simulink model "ES100A_SysStMod"  (R2013b)
settings: Solver=ode45  StartTime=0.0  StopTime=10  FixedStep=0.002  RelTol=1e-3
undefined symbols (not defined in the file): ELECGLBPRM_STRTUPSTTMPLMONININTESTCMPL_CNT_U08, sigbuilder_block, SysSt1, SYSSTMODPRSNTSTDI_CNT_U16, SYSSTMODPRSNTSTENA_CNT_U16, SYSSTMODPRSNTSTOFF_CNT_U16, SYSSTMODPRSNTSTWRMININ_CNT_U16
libraries: simulink x2
settings Model: Creator=pz79n7  LastModifiedBy=nzg49t
settings Model: ModifiedHistory=|
  | 05JN13: ES-10B Revision 011.  Added PStep/NStep counter (shown in red)
  | and calibrations to support.  This is in the block entitled "Safety Check" and
  | impacts NTC 0CB.  This change is in support of anomaly #5108.
  | 
  | 01JL13: ES-10B Revision 012.  Added note inside block "Determine Next State"
  | to clearly indicate that the state of the TOD signal is to be logic LOW when
  | switching is stopped.
  | 
  | 25JA15: ES-10B Revision 014 - Added links from Model to the FR document
  | 
  | 25JA15: ES-10B Revision 015 - Removed redundant check logic as it is no longer
  | needed based on new shutdown design placed into ES-34B.  Removed output
  | SysCSystemState and NTC 0CB.
settings DataIOCC: SignalLoggingSaveFormat=ModelDataLogs
settings OptimizationCC: ExpressionDepthLimit=2147483647
settings DebuggingCC: FcnCallInpInsideContextMsg=UseLocalSettings  StateNameClashWarn=warning
settings GRTTargetCC: CombineOutputUpdateFcns=off  GRTInterface=on

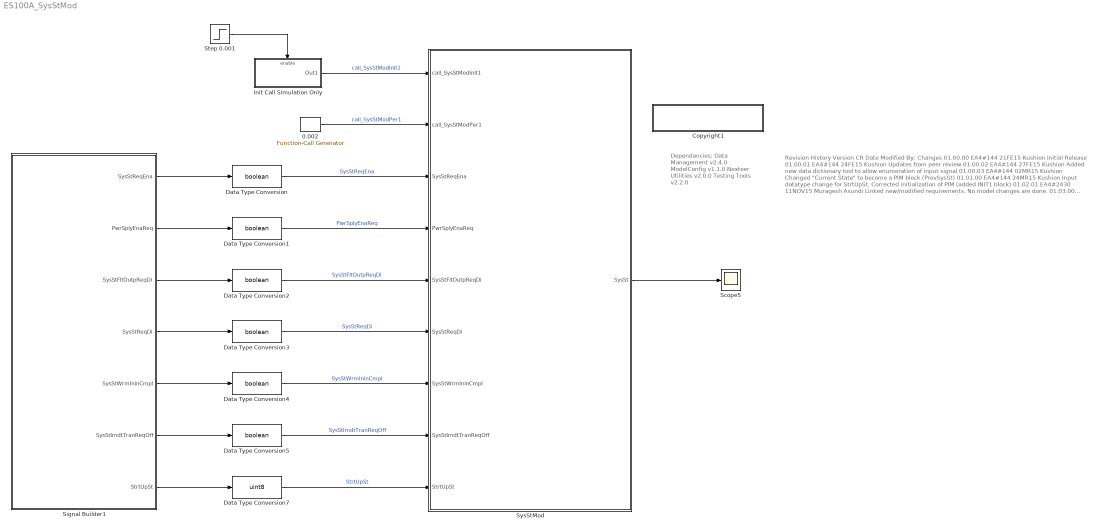
== system ES100A_SysStMod ==
  note: Revision History
      |
      | Version		CR			Date 		Modified By: 		Changes
      | 01.00.00 	EA4#144	21FE15		Kushion			Initial Release
      | 01.00.01		EA4#144       24FE15		Kushion			Updates from peer review
      | 01.00.02        EA4#144	27FE15		Kushion			Added new data dictionary tool to allow enumeration of input signal
      | 01.00.03		EA4#144	02MR15		Kushion			Changed "Current State" to become a PIM block (PrevSysSt)
      | 01.01.00	       EA4#144       24MR15        Kushion                 Input datatype change for StrtUpSt.  Corrected initialization of PIM (added INIT1 block)
      | 01.02.01        EA4#2430     11NOV15     Muragesh Asundi   Linked new/modified requirements. No model changes are done.
      | 01.03.00		EA4#4826	31MAR16	Kumaraswamy	Updated SysStReqEn => SysStReqEna, PwrSplyEnReq=> PwrSplyEnaReq to comply with
      | 													AUTOSAR Naming convention
  note: Dependancies:
      |    Data Management v2.4.0
      |    ModelConfig v1.1.0
      |    Nexteer Utilities v2.0.0
      |    Testing Tools v2.2.0
  0.002 : simulink/Ports & Subsystems/Function-Call Generator  sample_time=0.002  numberOfIterations=1
  Copyright1 : Subsystem  Description=|  mask(Copyright Information){none=on}
      | Copyright info block.                                               
      |                                                                     
      | Place copyright information at the top of every subsystem in design.
      mask prompts: none "No parameters"
      mask help: Place copyright information at the top of every subsystem in design.
      mask Display:
      | NxtrConf = 'Nexteer Confidential';
      | 
      | sys = bdroot; %handle for the current model ("system")
      | first = get_param(sys,'Created');
      | if(isempty(first))
      |     first = datestr(now,'yyyy');
      | else
      |     first = first(end-3:end);  %year is last four digits
      | end
      | 
      | last = get_param(sys,'LastModifiedDate');
      | if isempty(last)
      |     last = datestr(now,'yyyy');
      | else
      |     last = last(end-3:end);
      | end
      | 
      | if strcmp(first,last)
      |     fprintf('%s\nCopyright  %s Nexteer',NxtrConf,first);
      | else
      |     fprintf('%s\n%s%s-%s Nexteer',NxtrConf,char(169),first,last);
      | end
  Data Type Conversion : DataTypeConversion  Priority=1  OutDataTypeStr=boolean
  Data Type Conversion1 : DataTypeConversion  Priority=2  OutDataTypeStr=boolean
  Data Type Conversion2 : DataTypeConversion  Priority=3  OutDataTypeStr=boolean
  Data Type Conversion3 : DataTypeConversion  Priority=4  OutDataTypeStr=boolean
  Data Type Conversion4 : DataTypeConversion  Priority=5  OutDataTypeStr=boolean
  Data Type Conversion5 : DataTypeConversion  OutDataTypeStr=boolean
  Data Type Conversion7 : DataTypeConversion  OutDataTypeStr=uint8
  Init Call Simulation Only : Subsystem  TreatAsAtomicUnit=on
  Scope5 : Scope
      settings: TimeRange=10  YMin=-1  SaveName=ScopeData5  MaxDataPoints=10000
  Signal Builder1 : Subsystem  Tag=STV Subsys  LoadFcn=sigbuilder_block('load');  StartFcn=sigbuilder_block('start');  StopFcn=sigbuilder_block('stop');  ClipboardFcn=sigbuilder_block('clipboard');  mask(Sigbuilder block){}
      mask help: Create and generate interchangeable groups of signals whose waveforms are piecewise linear.
      mask init:
      | if ~strcmp(get_param(bdroot(gcbh),'SimulationStatus'),'stopped') tuvar = sigbuilder_block('maskInit'); end
      settings: CopyFcn=sigbuilder_block('copy');  DeleteFcn=sigbuilder_block('delete');  ModelCloseFcn=sigbuilder_block('modelClose');  PreSaveFcn=sigbuilder_block('preSave');  PauseFcn=sigbuilder_block('pause')  ContinueFcn=sigbuilder_block('continue')  NameChangeFcn=sigbuilder_block('namechange');  OpenFcn=sigbuilder_block('open',[1464 -138.75 381 502.5 ]);  CloseFcn=sigbuilder_block('close');
      mask Display: plot(0,0,100,100,[10,10,40,40,10],[80,20,20,80,80],[40,10],[50,50], [40,27,10],[65,72,56],[40,25,25,10],[28,28,43,43]);
  Step 0.001 : Step  Time=0.001  Before=1  After=0  SampleTime=0
  SysStMod : Subsystem  RequirementInfo={'linktype_rmi_doors' '0000cf67 (/E-STEER Core/SubSystem Specifications/Electrical Actuator/Control Module/FDD Module Requirements/EA4/ES100A_SysStMod_1)' '#ES100A_72' 'true' 'REQ: ES100A_72' '' ; 'linktype_rmi_doors' '0000cf67 (/E-STEER Core/SubSystem Specifications/Electrical Actuator/Control Module/FDD Module Requirements/EA4/ES100A_SysStMod_1)' '#ES100A_80' 'true' 'REQ: ES100A_80' '' } %GIDa_7525e75c_09f9_4f81_91ae_9ba7a4b2fbd2
  wires:
  SysStMod/1(SysSt) -> Scope5/1
  Signal Builder1/1(SysStReqEna) -> Data Type Conversion/1
  Signal Builder1/2(PwrSplyEnaReq) -> Data Type Conversion1/1
  Signal Builder1/3(SysStFltOutpReqDi) -> Data Type Conversion2/1
  Signal Builder1/4(SysStReqDi) -> Data Type Conversion3/1
  Signal Builder1/5(SysStWrmIninCmpl) -> Data Type Conversion4/1
  Signal Builder1/6(SysStImdtTranReqOff) -> Data Type Conversion5/1
  Data Type Conversion/1 -> SysStMod/3(SysStReqEna)  "SysStReqEna"
  Data Type Conversion1/1 -> SysStMod/4(PwrSplyEnaReq)  "PwrSplyEnaReq"
  Data Type Conversion2/1 -> SysStMod/5(SysStFltOutpReqDi)  "SysStFltOutpReqDi"
  Data Type Conversion3/1 -> SysStMod/6(SysStReqDi)  "SysStReqDi"
  Data Type Conversion4/1 -> SysStMod/7(SysStWrmIninCmpl)  "SysStWrmIninCmpl"
  Data Type Conversion5/1 -> SysStMod/8(SysStImdtTranReqOff)  "SysStImdtTranReqOff"
  Signal Builder1/7(StrtUpSt) -> Data Type Conversion7/1
  0.002/1 -> SysStMod/2(call_SysStModPer1)  "call_SysStModPer1"
  Data Type Conversion7/1 -> SysStMod/9(StrtUpSt)  "StrtUpSt"
  Init Call Simulation Only/1(Out1) -> SysStMod/1(call_SysStModInit1)  "call_SysStModInit1"
  Step 0.001/1 -> Init Call Simulation Only/Enable

== system ES100A_SysStMod/Copyright1 ==

== system ES100A_SysStMod/Init Call Simulation Only ==
  Enable : EnablePort
  0.001 : simulink/Ports & Subsystems/Function-Call Generator  sample_time=0.001  numberOfIterations=1
  Out1 : Outport
  wires:
  0.001/1 -> Out1/1

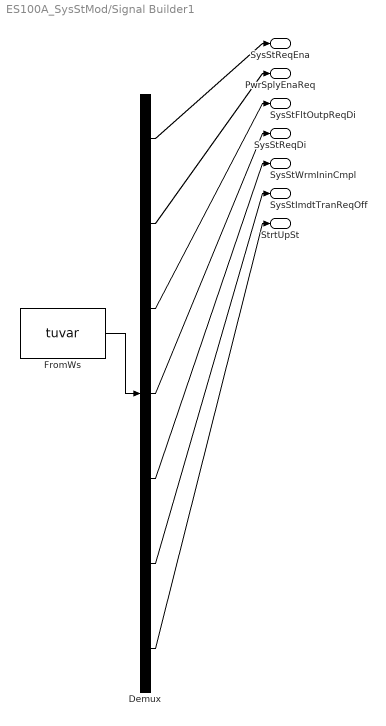
== system ES100A_SysStMod/Signal Builder1 ==
  Demux : Demux  Tag=STV Demux  Outputs=7
  FromWs : FromWorkspace  Tag=STV FromWs  VariableName=tuvar  SampleTime=0.002
      SigBuilderData=|
      | common.afterFinalStr = 'Extrapolate'
      | common.sampleTime = '0.002'
      | dataSet(1).timeRange = [0 10]
      | dataSet(1).name = 'Normal Start up to Enable'
      | dataSet(2).timeRange = [0 10]
      | dataSet(2).name = 'Confirm no ENABLE until WI is complete'
      | dataSet(3).timeRange = [0 10]
      | dataSet(3).name = 'Normal cycle - WI, Operate, Disable, OFF'
      | dataSet(4).timeRange = [0 10]
      | dataSet(4).name = 'While in WI, Change ReqDI, no changem Cgange Fault, DIS'
      | dataSet(5).timeRange = [0 10]
      | dataSet(5).name = 'Rapid shutdown while in operate state'
      | dataSet(6).timeRange = [0 10]
      | dataSet(6).name = 'Quick Ignition (assumed prior to TOD off)'
      | dataSet(7).timeRange = [0 10]
      | dataSet(7).name = 'Failure in warm init prior to temporal monitor completing'
      | dataSet(8).timeRange = [0 10]
      | dataSet(8).name = 'Immediate request from Reset or FBL'
      | sbobj.Groups(1).Name = 'Normal Start up to Enable'
      | sbobj.Groups(1).Signals(1).Name = 'SysStReqEna'
      | sbobj.Groups(1).Signals(1).XData = [0 2 2 6 6 10]
      | sbobj.Groups(1).Signals(1).YData = [0 0 1 1 0 0]
      | sbobj.Groups(1).Signals(2).Name = 'PwrSplyEnaReq'
      | sbobj.Groups(1).Signals(2).XData = [0 6 6 10]
      | sbobj.Groups(1).Signals(2).YData = [1 1 0 0]
      | sbobj.Groups(1).Signals(3).Name = 'SysStFltOutpReqDi'
      | sbobj.Groups(1).Signals(3).XData = [0 4 6 10]
      | sbobj.Groups(1).Signals(3).YData = [0 0 0 0]
      | sbobj.Groups(1).Signals(4).Name = 'SysStReqDi'
      | sbobj.Groups(1).Signals(4).XData = [0 4 6 10]
      | sbobj.Groups(1).Signals(4).YData = [0 0 0 0]
      | sbobj.Groups(1).Signals(5).Name = 'SysStWrmIninCmpl'
      | sbobj.Groups(1).Signals(5).XData = [0 1 1 6 6 10]
      | sbobj.Groups(1).Signals(5).YData = [0 0 1 1 0 0]
      | sbobj.Groups(1).Signals(6).Name = 'SysStImdtTranReqOff'
      | sbobj.Groups(1).Signals(6).XData = [0 4 6 10]
      | sbobj.Groups(1).Signals(6).YData = [0 0 0 0]
      | sbobj.Groups(1).Signals(7).Name = 'StrtUpSt'
      | sbobj.Groups(1).Signals(7).XData = [0 0.5 0.5 6 6 10]
      | sbobj.Groups(1).Signals(7).YData = [1 1 3 3 1 1]
      | sbobj.Groups(2).Name = 'Confirm no ENABLE until WI is complete'
      | sbobj.Groups(2).Signals(1).Name = 'SysStReqEna'
      | sbobj.Groups(2).Signals(1).XData = [0 0.5 0.5 6 6 10]
      | sbobj.Groups(2).Signals(1).YData = [0 0 1 1 0 0]
      | sbobj.Groups(2).Signals(2).Name = 'PwrSplyEnaReq'
      | sbobj.Groups(2).Signals(2).XData = [0 6 6 10]
      | sbobj.Groups(2).Signals(2).YData = [1 1 0 0]
      | sbobj.Groups(2).Signals(3).Name = 'SysStFltOutpReqDi'
      | sbobj.Groups(2).Signals(3).XData = [0 4 6 10]
      | sbobj.Groups(2).Signals(3).YData = [0 0 0 0]
      | sbobj.Groups(2).Signals(4).Name = 'SysStReqDi'
      | sbobj.Groups(2).Signals(4).XData = [0 8 8 10]
      | sbobj.Groups(2).Signals(4).YData = [0 0 1 1]
      | sbobj.Groups(2).Signals(5).Name = 'SysStWrmIninCmpl'
      | sbobj.Groups(2).Signals(5).XData = [0 1 1 6 6 10]
      | sbobj.Groups(2).Signals(5).YData = [0 0 1 1 0 0]
      | sbobj.Groups(2).Signals(6).Name = 'SysStImdtTranReqOff'
      | sbobj.Groups(2).Signals(6).XData = [0 4 6 10]
      | sbobj.Groups(2).Signals(6).YData = [0 0 0 0]
      | sbobj.Groups(2).Signals(7).Name = 'StrtUpSt'
      | sbobj.Groups(2).Signals(7).XData = [0 0.5 0.5 6 6 10]
      | sbobj.Groups(2).Signals(7).YData = [1 1 3 3 1 1]
      | sbobj.Groups(3).Name = 'Normal cycle - WI, Operate, Disable, OFF'
      | sbobj.Groups(3).Signals(1).Name = 'SysStReqEna'
      | sbobj.Groups(3).Signals(1).XData = [0 2 2 6 6 10]
      | sbobj.Groups(3).Signals(1).YData = [0 0 1 1 0 0]
      | sbobj.Groups(3).Signals(2).Name = 'PwrSplyEnaReq'
      | sbobj.Groups(3).Signals(2).XData = [0 9 9 10]
      | sbobj.Groups(3).Signals(2).YData = [1 1 0 0]
      | sbobj.Groups(3).Signals(3).Name = 'SysStFltOutpReqDi'
      | sbobj.Groups(3).Signals(3).XData = [0 7.5 10]
      | sbobj.Groups(3).Signals(3).YData = [0 0 0]
      | sbobj.Groups(3).Signals(4).Name = 'SysStReqDi'
      | sbobj.Groups(3).Signals(4).XData = [0 7.5 7.5 10]
      | sbobj.Groups(3).Signals(4).YData = [0 0 1 1]
      | sbobj.Groups(3).Signals(5).Name = 'SysStWrmIninCmpl'
      | sbobj.Groups(3).Signals(5).XData = [0 1 1 10]
      | sbobj.Groups(3).Signals(5).YData = [0 0 1 1]
      | sbobj.Groups(3).Signals(6).Name = 'SysStImdtTranReqOff'
      | sbobj.Groups(3).Signals(6).XData = [0 4 6 10]
      | sbobj.Groups(3).Signals(6).YData = [0 0 0 0]
      | sbobj.Groups(3).Signals(7).Name = 'StrtUpSt'
      | sbobj.Groups(3).Signals(7).XData = [0 0.5 0.5 10]
      | sbobj.Groups(3).Signals(7).YData = [1 1 3 3]
      | sbobj.Groups(4).Name = 'While in WI, Change ReqDI, no changem Cgange Fault, DIS'
      | sbobj.Groups(4).Signals(1).Name = 'SysStReqEna'
      | sbobj.Groups(4).Signals(1).XData = [0 3 10]
      | sbobj.Groups(4).Signals(1).YData = [0 0 0]
      | sbobj.Groups(4).Signals(2).Name = 'PwrSplyEnaReq'
      | sbobj.Groups(4).Signals(2).XData = [0 9 9 10]
      | sbobj.Groups(4).Signals(2).YData = [1 1 0 0]
      | sbobj.Groups(4).Signals(3).Name = 'SysStFltOutpReqDi'
      | sbobj.Groups(4).Signals(3).XData = [0 5 5 10]
      | sbobj.Groups(4).Signals(3).YData = [0 0 1 1]
      | sbobj.Groups(4).Signals(4).Name = 'SysStReqDi'
      | sbobj.Groups(4).Signals(4).XData = [0 3 3 10]
      | sbobj.Groups(4).Signals(4).YData = [0 0 1 1]
      | sbobj.Groups(4).Signals(5).Name = 'SysStWrmIninCmpl'
      | sbobj.Groups(4).Signals(5).XData = [0 1 1 10]
      | sbobj.Groups(4).Signals(5).YData = [0 0 1 1]
      | sbobj.Groups(4).Signals(6).Name = 'SysStImdtTranReqOff'
      | sbobj.Groups(4).Signals(6).XData = [0 4 6 10]
      | sbobj.Groups(4).Signals(6).YData = [0 0 0 0]
      | sbobj.Groups(4).Signals(7).Name = 'StrtUpSt'
      | sbobj.Groups(4).Signals(7).XData = [0 0.5 0.5 10]
      | sbobj.Groups(4).Signals(7).YData = [1 1 3 3]
      | sbobj.Groups(5).Name = 'Rapid shutdown while in operate state'
      | sbobj.Groups(5).Signals(1).Name = 'SysStReqEna'
      | sbobj.Groups(5).Signals(1).XData = [0 2 2 10]
      | sbobj.Groups(5).Signals(1).YData = [0 0 1 1]
      | sbobj.Groups(5).Signals(2).Name = 'PwrSplyEnaReq'
      | sbobj.Groups(5).Signals(2).XData = [0 9 9 10]
      | sbobj.Groups(5).Signals(2).YData = [1 1 0 0]
      | sbobj.Groups(5).Signals(3).Name = 'SysStFltOutpReqDi'
      | sbobj.Groups(5).Signals(3).XData = [0 4 4 10]
      | sbobj.Groups(5).Signals(3).YData = [0 0 1 1]
      | sbobj.Groups(5).Signals(4).Name = 'SysStReqDi'
      | sbobj.Groups(5).Signals(4).XData = [0 4 4 10]
      | sbobj.Groups(5).Signals(4).YData = [0 0 1 1]
      | sbobj.Groups(5).Signals(5).Name = 'SysStWrmIninCmpl'
      | sbobj.Groups(5).Signals(5).XData = [0 1 1 10]
      | sbobj.Groups(5).Signals(5).YData = [0 0 1 1]
      | sbobj.Groups(5).Signals(6).Name = 'SysStImdtTranReqOff'
      | sbobj.Groups(5).Signals(6).XData = [0 4 6 10]
      | sbobj.Groups(5).Signals(6).YData = [0 0 0 0]
      | sbobj.Groups(5).Signals(7).Name = 'StrtUpSt'
      | sbobj.Groups(5).Signals(7).XData = [0 0.5 0.5 10]
      | sbobj.Groups(5).Signals(7).YData = [1 1 3 3]
      | sbobj.Groups(6).Name = 'Quick Ignition (assumed prior to TOD off)'
      | sbobj.Groups(6).Signals(1).Name = 'SysStReqEna'
      | sbobj.Groups(6).Signals(1).XData = [0 1.5 1.5 4 4 5.5 5.5 10]
      | sbobj.Groups(6).Signals(1).YData = [0 0 1 1 0 0 1 1]
      | sbobj.Groups(6).Signals(2).Name = 'PwrSplyEnaReq'
      | sbobj.Groups(6).Signals(2).XData = [0 4 4 5.5 5.5 10]
      | sbobj.Groups(6).Signals(2).YData = [1 1 0 0 1 1]
      | sbobj.Groups(6).Signals(3).Name = 'SysStFltOutpReqDi'
      | sbobj.Groups(6).Signals(3).XData = [0 5 10]
      | sbobj.Groups(6).Signals(3).YData = [0 0 0]
      | sbobj.Groups(6).Signals(4).Name = 'SysStReqDi'
      | sbobj.Groups(6).Signals(4).XData = [0 5 5 10]
      | sbobj.Groups(6).Signals(4).YData = [0 0 1 1]
      | sbobj.Groups(6).Signals(5).Name = 'SysStWrmIninCmpl'
      | sbobj.Groups(6).Signals(5).XData = [0 1 1 10]
      | sbobj.Groups(6).Signals(5).YData = [0 0 1 1]
      | sbobj.Groups(6).Signals(6).Name = 'SysStImdtTranReqOff'
      | sbobj.Groups(6).Signals(6).XData = [0 4 6 10]
      | sbobj.Groups(6).Signals(6).YData = [0 0 0 0]
      | sbobj.Groups(6).Signals(7).Name = 'StrtUpSt'
      | sbobj.Groups(6).Signals(7).XData = [0 0.5 0.5 10]
      | sbobj.Groups(6).Signals(7).YData = [1 1 3 3]
      | sbobj.Groups(7).Name = 'Failure in warm init prior to temporal monitor completing'
      | sbobj.Groups(7).Signals(1).Name = 'SysStReqEna'
      | sbobj.Groups(7).Signals(1).XData = [0 0.5 0.5 4 5.5 10]
      | sbobj.Groups(7).Signals(1).YData = [0 0 1 1 1 1]
      | sbobj.Groups(7).Signals(2).Name = 'PwrSplyEnaReq'
      | sbobj.Groups(7).Signals(2).XData = [0 4 10]
      | sbobj.Groups(7).Signals(2).YData = [1 1 1]
      | sbobj.Groups(7).Signals(3).Name = 'SysStFltOutpReqDi'
      | sbobj.Groups(7).Signals(3).XData = [0 1.5 1.5 10]
      | sbobj.Groups(7).Signals(3).YData = [0 0 1 1]
      | sbobj.Groups(7).Signals(4).Name = 'SysStReqDi'
      | sbobj.Groups(7).Signals(4).XData = [0 1.5 1.5 10]
      | sbobj.Groups(7).Signals(4).YData = [0 0 1 1]
      | sbobj.Groups(7).Signals(5).Name = 'SysStWrmIninCmpl'
      | sbobj.Groups(7).Signals(5).XData = [0 4 4 10]
      | sbobj.Groups(7).Signals(5).YData = [0 0 1 1]
      | sbobj.Groups(7).Signals(6).Name = 'SysStImdtTranReqOff'
      | sbobj.Groups(7).Signals(6).XData = [0 4 6 10]
      | sbobj.Groups(7).Signals(6).YData = [0 0 0 0]
      | sbobj.Groups(7).Signals(7).Name = 'StrtUpSt'
      | sbobj.Groups(7).Signals(7).XData = [0 2.5 2.5 10]
      | sbobj.Groups(7).Signals(7).YData = [1 1 3 3]
      | sbobj.Groups(8).Name = 'Immediate request from Reset or FBL'
      | sbobj.Groups(8).Signals(1).Name = 'SysStReqEna'
      | sbobj.Groups(8).Signals(1).XData = [0 1.5 1.5 4 5.5 10]
      | sbobj.Groups(8).Signals(1).YData = [0 0 1 1 1 1]
      | sbobj.Groups(8).Signals(2).Name = 'PwrSplyEnaReq'
      | sbobj.Groups(8).Signals(2).XData = [0 4 10]
      | sbobj.Groups(8).Signals(2).YData = [1 1 1]
      | sbobj.Groups(8).Signals(3).Name = 'SysStFltOutpReqDi'
      | sbobj.Groups(8).Signals(3).XData = [0 1.5 10]
      | sbobj.Groups(8).Signals(3).YData = [0 0 0]
      | sbobj.Groups(8).Signals(4).Name = 'SysStReqDi'
      | sbobj.Groups(8).Signals(4).XData = [0 1.5 10]
      | sbobj.Groups(8).Signals(4).YData = [0 0 0]
      | sbobj.Groups(8).Signals(5).Name = 'SysStWrmIninCmpl'
      | sbobj.Groups(8).Signals(5).XData = [0 1 1 10]
      | sbobj.Groups(8).Signals(5).YData = [0 0 1 1]
      | sbobj.Groups(8).Signals(6).Name = 'SysStImdtTranReqOff'
      | sbobj.Groups(8).Signals(6).XData = [0 4 4 8 8 10]
      | sbobj.Groups(8).Signals(6).YData = [0 0 1 1 0 0]
      | sbobj.Groups(8).Signals(7).Name = 'StrtUpSt'
      | sbobj.Groups(8).Signals(7).XData = [0 0.5 0.5 10]
      | sbobj.Groups(8).Signals(7).YData = [1 1 3 3]
  SysStReqEna : Outport  Tag=STV Outport
  PwrSplyEnaReq : Outport  Tag=STV Outport  Port=2
  SysStFltOutpReqDi : Outport  Tag=STV Outport  Port=3
  SysStReqDi : Outport  Tag=STV Outport  Port=4
  SysStWrmIninCmpl : Outport  Tag=STV Outport  Port=5
  SysStImdtTranReqOff : Outport  Tag=STV Outport  Port=6
  StrtUpSt : Outport  Tag=STV Outport  Port=7
  wires:
  FromWs/1 -> Demux/1
  Demux/1 -> SysStReqEna/1
  Demux/2 -> PwrSplyEnaReq/1
  Demux/3 -> SysStFltOutpReqDi/1
  Demux/4 -> SysStReqDi/1
  Demux/5 -> SysStWrmIninCmpl/1
  Demux/6 -> SysStImdtTranReqOff/1
  Demux/7 -> StrtUpSt/1

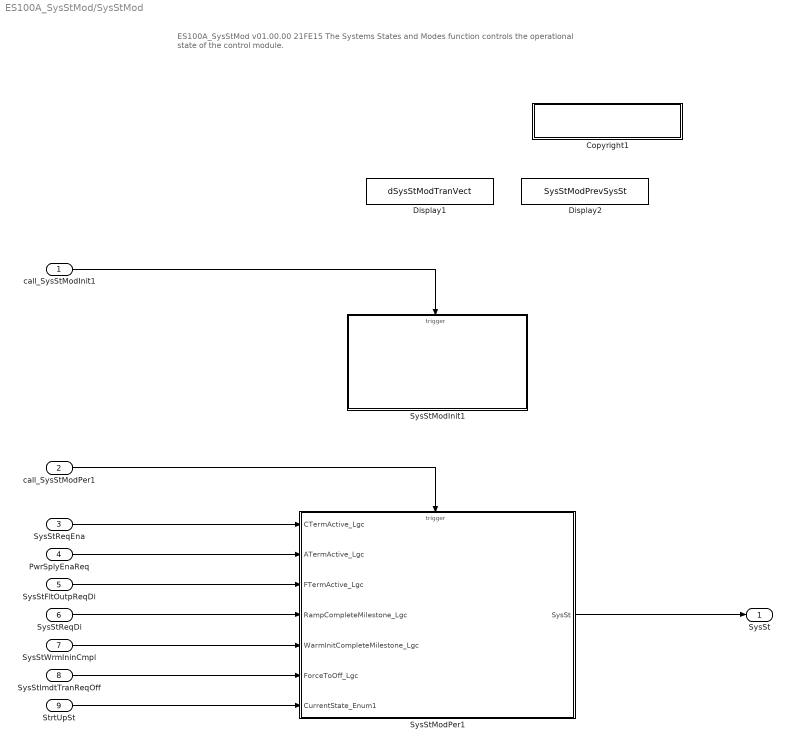
== system ES100A_SysStMod/SysStMod ==
  note: ES100A_SysStMod
      | v01.00.00  21FE15
      |
      | The Systems States and Modes function controls the operational state of the control module.
  call_SysStModInit1 : Inport  RequirementInfo={} %GIDa_70abc33c_fbc6_4489_97a9_d53097d440a5
  call_SysStModPer1 : Inport  RequirementInfo={} %GIDa_247d166b_4762_4bdb_9ac9_c1341da72383  Port=2
  SysStReqEna : Inport  RequirementInfo={'linktype_rmi_doors' '0000cf67 (/E-STEER Core/SubSystem Specifications/Electrical Actuator/Control Module/FDD Module Requirements/EA4/ES100A_SysStMod_1)' '#ES100A_66' 'true' 'REQ: ES100A_66' '' } %GIDa_6d7fad2b_a94e_495f_a571_8467ce8a9fcd  Port=3
  PwrSplyEnaReq : Inport  RequirementInfo={} %GIDa_9df901b6_084e_4a14_9c60_1b090c551106  Port=4
  SysStFltOutpReqDi : Inport  RequirementInfo={'linktype_rmi_doors' '0000cf67 (/E-STEER Core/SubSystem Specifications/Electrical Actuator/Control Module/FDD Module Requirements/EA4/ES100A_SysStMod_1)' '#ES100A_65' 'true' 'REQ: ES100A_65' '' } %GIDa_df7e7c0b_c10a_4285_849c_6ef5f31a5559  Port=5
  SysStReqDi : Inport  RequirementInfo={'linktype_rmi_doors' '0000cf67 (/E-STEER Core/SubSystem Specifications/Electrical Actuator/Control Module/FDD Module Requirements/EA4/ES100A_SysStMod_1)' '#ES100A_67' 'true' 'REQ: ES100A_67' '' } %GIDa_35b356da_e40e_4e97_938f_a1c7151ed980  Port=6
  SysStWrmIninCmpl : Inport  RequirementInfo={'linktype_rmi_doors' '0000cf67 (/E-STEER Core/SubSystem Specifications/Electrical Actuator/Control Module/FDD Module Requirements/EA4/ES100A_SysStMod_1)' '#ES100A_68' 'true' 'REQ: ES100A_68' '' } %GIDa_4d13480c_622e_4454_9875_58918840b823  Port=7
  SysStImdtTranReqOff : Inport  RequirementInfo={'linktype_rmi_doors' '0000cf67 (/E-STEER Core/SubSystem Specifications/Electrical Actuator/Control Module/FDD Module Requirements/EA4/ES100A_SysStMod_1)' '#ES100A_69' 'true' 'REQ: ES100A_69' '' } %GIDa_6f7c4454_acb4_41a2_b8b6_4cde36a838aa  Port=8
  StrtUpSt : Inport  RequirementInfo={'linktype_rmi_doors' '0000cf67 (/E-STEER Core/SubSystem Specifications/Electrical Actuator/Control Module/FDD Module Requirements/EA4/ES100A_SysStMod_1)' '#ES100A_70' 'true' 'REQ: ES100A_70' '' } %GIDa_9e13d533_05b6_4979_b484_35e385ca2454  Port=9
  Copyright1 : Subsystem  Description=|  mask(Copyright Information){none=on}
      | Copyright info block.                                               
      |                                                                     
      | Place copyright information at the top of every subsystem in design.
      mask prompts: none "No parameters"
      mask help: Place copyright information at the top of every subsystem in design.
      mask Display:
      | NxtrConf = 'Nexteer Confidential';
      | 
      | sys = bdroot; %handle for the current model ("system")
      | first = get_param(sys,'Created');
      | if(isempty(first))
      |     first = datestr(now,'yyyy');
      | else
      |     first = first(end-3:end);  %year is last four digits
      | end
      | 
      | last = get_param(sys,'LastModifiedDate');
      | if isempty(last)
      |     last = datestr(now,'yyyy');
      | else
      |     last = last(end-3:end);
      | end
      | 
      | if strcmp(first,last)
      |     fprintf('%s\nCopyright  %s Nexteer',NxtrConf,first);
      | else
      |     fprintf('%s\n%s%s-%s Nexteer',NxtrConf,char(169),first,last);
      | end
  Display1 : DataStoreMemory  DataStoreName=dSysStModTranVect  ReadBeforeWriteMsg=warning  WriteAfterWriteMsg=warning  WriteAfterReadMsg=warning  OutDataTypeStr=uint16  StateMustResolveToSignalObject=on
  Display2 : DataStoreMemory  DataStoreName=SysStModPrevSysSt  OutDataTypeStr=uint16  StateMustResolveToSignalObject=on
  SysStModInit1 : Subsystem
  SysStModPer1 : Subsystem  RequirementInfo={'linktype_rmi_doors' '0000cf67 (/E-STEER Core/SubSystem Specifications/Electrical Actuator/Control Module/FDD Module Requirements/EA4/ES100A_SysStMod_1)' '#ES100A_77' 'true' 'REQ: ES100A_77' '' ; 'linktype_rmi_doors' '0000cf67 (/E-STEER Core/SubSystem Specifications/Electrical Actuator/Control Module/FDD Module Requirements/EA4/ES100A_SysStMod_1)' '#ES100A_80' 'true' 'REQ: ES100A_80' '' } %GIDa_993dbca0_2899_4b0b_9f81_f621807feeb3
  SysSt : Outport  RequirementInfo={'linktype_rmi_doors' '0000cf67 (/E-STEER Core/SubSystem Specifications/Electrical Actuator/Control Module/FDD Module Requirements/EA4/ES100A_SysStMod_1)' '#ES100A_51' 'true' 'REQ: ES100A_51' '' } %GIDa_1bed07cb_a357_4d89_8b33_d3411b40c752
  wires:
  SysStReqEna/1 -> SysStModPer1/1(CTermActive_Lgc)
  PwrSplyEnaReq/1 -> SysStModPer1/2(ATermActive_Lgc)
  SysStFltOutpReqDi/1 -> SysStModPer1/3(FTermActive_Lgc)
  SysStReqDi/1 -> SysStModPer1/4(RampCompleteMilestone_Lgc)
  SysStWrmIninCmpl/1 -> SysStModPer1/5(WarmInitCompleteMilestone_Lgc)
  SysStImdtTranReqOff/1 -> SysStModPer1/6(ForceToOff_Lgc)
  StrtUpSt/1 -> SysStModPer1/7(CurrentState_Enum1)
  SysStModPer1/1(SysSt) -> SysSt/1
  call_SysStModPer1/1 -> SysStModPer1/Trigger
  call_SysStModInit1/1 -> SysStModInit1/Trigger

== system ES100A_SysStMod/SysStMod/Copyright1 ==

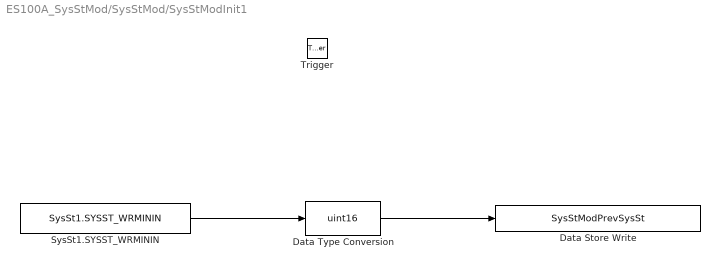
== system ES100A_SysStMod/SysStMod/SysStModInit1 ==
  Trigger : TriggerPort  TriggerType=function-call  PortDimensions=1
  Data Store Write : DataStoreWrite  RequirementInfo={'linktype_rmi_doors' '0000cf67 (/E-STEER Core/SubSystem Specifications/Electrical Actuator/Control Module/FDD Module Requirements/EA4/ES100A_SysStMod_1)' '#ES100A_87' 'true' 'REQ: ES100A_87' '' } %GIDa_615beef4_a9b1_4f63_b9c7_03e636d72f5d  DataStoreName=SysStModPrevSysSt
  Data Type Conversion : DataTypeConversion  OutDataTypeStr=uint16
  SysSt1.SYSST_WRMININ : Constant  RequirementInfo={'linktype_rmi_doors' '0000cf67 (/E-STEER Core/SubSystem Specifications/Electrical Actuator/Control Module/FDD Module Requirements/EA4/ES100A_SysStMod_1)' '#ES100A_87' 'true' 'REQ: ES100A_87' '' } %GIDa_171fb50a_baa0_4c2d_a177_2860f6d4deea  Value=SysSt1.SYSST_WRMININ
  wires:
  SysSt1.SYSST_WRMININ/1 -> Data Type Conversion/1
  Data Type Conversion/1 -> Data Store Write/1

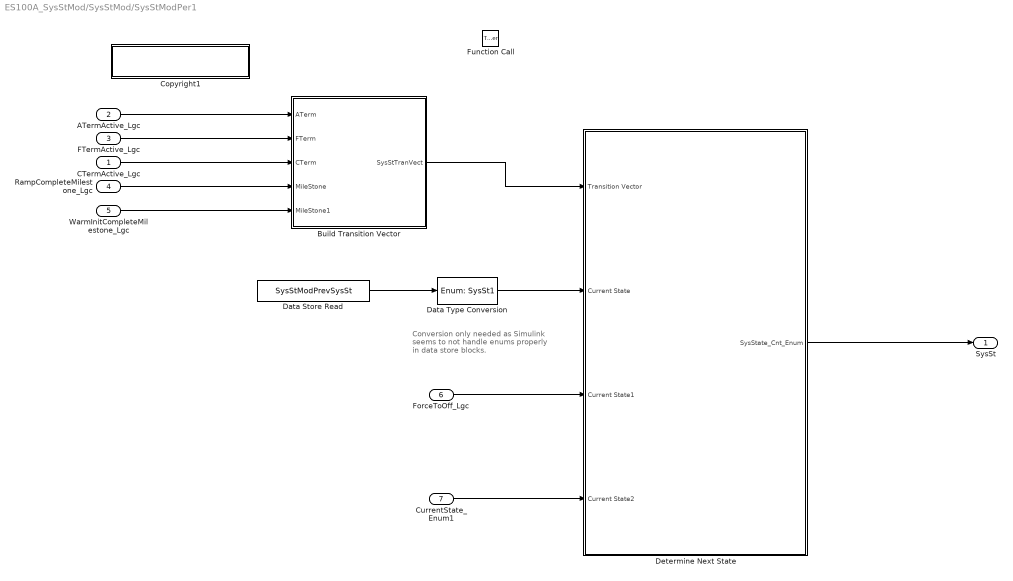
== system ES100A_SysStMod/SysStMod/SysStModPer1 ==
  note: Conversion only needed as Simulink
      | seems to not handle enums properly
      | in data store blocks.
  CTermActive_Lgc : Inport  RequirementInfo={'linktype_rmi_doors' '0000cf67 (/E-STEER Core/SubSystem Specifications/Electrical Actuator/Control Module/FDD Module Requirements/EA4/ES100A_SysStMod_1)' '#ES100A_66' 'true' 'REQ: ES100A_66' '' } %GIDa_6d7fad2b_a94e_495f_a571_8467ce8a9fcd
  ATermActive_Lgc : Inport  RequirementInfo={} %GIDa_9df901b6_084e_4a14_9c60_1b090c551106  Port=2
  FTermActive_Lgc : Inport  RequirementInfo={'linktype_rmi_doors' '0000cf67 (/E-STEER Core/SubSystem Specifications/Electrical Actuator/Control Module/FDD Module Requirements/EA4/ES100A_SysStMod_1)' '#ES100A_65' 'true' 'REQ: ES100A_65' '' } %GIDa_df7e7c0b_c10a_4285_849c_6ef5f31a5559  Port=3
  RampCompleteMilestone_Lgc : Inport  RequirementInfo={'linktype_rmi_doors' '0000cf67 (/E-STEER Core/SubSystem Specifications/Electrical Actuator/Control Module/FDD Module Requirements/EA4/ES100A_SysStMod_1)' '#ES100A_67' 'true' 'REQ: ES100A_67' '' } %GIDa_35b356da_e40e_4e97_938f_a1c7151ed980  Port=4
  WarmInitCompleteMilestone_Lgc : Inport  RequirementInfo={'linktype_rmi_doors' '0000cf67 (/E-STEER Core/SubSystem Specifications/Electrical Actuator/Control Module/FDD Module Requirements/EA4/ES100A_SysStMod_1)' '#ES100A_68' 'true' 'REQ: ES100A_68' '' } %GIDa_4d13480c_622e_4454_9875_58918840b823  Port=5
  ForceToOff_Lgc : Inport  RequirementInfo={'linktype_rmi_doors' '0000cf67 (/E-STEER Core/SubSystem Specifications/Electrical Actuator/Control Module/FDD Module Requirements/EA4/ES100A_SysStMod_1)' '#ES100A_69' 'true' 'REQ: ES100A_69' '' } %GIDa_6f7c4454_acb4_41a2_b8b6_4cde36a838aa  Port=6
  CurrentState_Enum1 : Inport  RequirementInfo={'linktype_rmi_doors' '0000cf67 (/E-STEER Core/SubSystem Specifications/Electrical Actuator/Control Module/FDD Module Requirements/EA4/ES100A_SysStMod_1)' '#ES100A_70' 'true' 'REQ: ES100A_70' '' } %GIDa_9e13d533_05b6_4979_b484_35e385ca2454  Port=7
  Function Call : TriggerPort  TriggerType=function-call  PortDimensions=1
  Build Transition Vector : Subsystem  RequirementInfo={'linktype_rmi_doors' '0000cf67 (/E-STEER Core/SubSystem Specifications/Electrical Actuator/Control Module/FDD Module Requirements/EA4/ES100A_SysStMod_1)' '#ES100A_73' 'true' 'REQ: ES100A_73' '' ; 'linktype_rmi_doors' '0000cf67 (/E-STEER Core/SubSystem Specifications/Electrical Actuator/Control Module/FDD Module Requirements/EA4/ES100A_SysStMod_1)' '#ES100A_76' 'true' 'REQ: ES100A_76' '' } %GIDa_2f89c87b_c7f4_45b5_8d21_7478fe3bd3c1
  Copyright1 : Subsystem  Description=|  mask(Copyright Information){none=on}
      | Copyright info block.                                               
      |                                                                     
      | Place copyright information at the top of every subsystem in design.
      mask prompts: none "No parameters"
      mask help: Place copyright information at the top of every subsystem in design.
      mask Display:
      | NxtrConf = 'Nexteer Confidential';
      | 
      | sys = bdroot; %handle for the current model ("system")
      | first = get_param(sys,'Created');
      | if(isempty(first))
      |     first = datestr(now,'yyyy');
      | else
      |     first = first(end-3:end);  %year is last four digits
      | end
      | 
      | last = get_param(sys,'LastModifiedDate');
      | if isempty(last)
      |     last = datestr(now,'yyyy');
      | else
      |     last = last(end-3:end);
      | end
      | 
      | if strcmp(first,last)
      |     fprintf('%s\nCopyright  %s Nexteer',NxtrConf,first);
      | else
      |     fprintf('%s\n%s%s-%s Nexteer',NxtrConf,char(169),first,last);
      | end
  Data Store Read : DataStoreRead  DataStoreName=SysStModPrevSysSt
  Data Type Conversion : DataTypeConversion  OutDataTypeStr=Enum: SysSt1
  Determine Next State : Subsystem  RequirementInfo={'linktype_rmi_doors' '0000cf67 (/E-STEER Core/SubSystem Specifications/Electrical Actuator/Control Module/FDD Module Requirements/EA4/ES100A_SysStMod_1)' '#ES100A_77' 'true' 'REQ: ES100A_77' '' ; 'linktype_rmi_doors' '0000cf67 (/E-STEER Core/SubSystem Specifications/Electrical Actuator/Control Module/FDD Module Requirements/EA4/ES100A_SysStMod_1)' '#ES100A_78' 'true' 'REQ: ES100A_78' '' } %GIDa_7bf8c2ea_37ec_4b7d_b11a_3048b84ef03b
  SysSt : Outport  RequirementInfo={'linktype_rmi_doors' '0000cf67 (/E-STEER Core/SubSystem Specifications/Electrical Actuator/Control Module/FDD Module Requirements/EA4/ES100A_SysStMod_1)' '#ES100A_51' 'true' 'REQ: ES100A_51' '' ; 'linktype_rmi_doors' '0000cf67 (/E-STEER Core/SubSystem Specifications/Electrical Actuator/Control Module/FDD Module Requirements/EA4/ES100A_SysStMod_1)' '#ES100A_32' 'true' 'REQ: ES100A_32' '' } %GIDa_1bed07cb_a357_4d89_8b33_d3411b40c752
  wires:
  Build Transition Vector/1(SysStTranVect) -> Determine Next State/1(Transition Vector)
  RampCompleteMilestone_Lgc/1 -> Build Transition Vector/4(MileStone)
  CurrentState_Enum1/1 -> Determine Next State/4(Current State2)
  CTermActive_Lgc/1 -> Build Transition Vector/3(CTerm)
  FTermActive_Lgc/1 -> Build Transition Vector/2(FTerm)
  Data Store Read/1 -> Data Type Conversion/1
  ATermActive_Lgc/1 -> Build Transition Vector/1(ATerm)
  ForceToOff_Lgc/1 -> Determine Next State/3(Current State1)
  WarmInitCompleteMilestone_Lgc/1 -> Build Transition Vector/5(MileStone1)
  Determine Next State/1(SysState_Cnt_Enum) -> SysSt/1
  Data Type Conversion/1 -> Determine Next State/2(Current State)

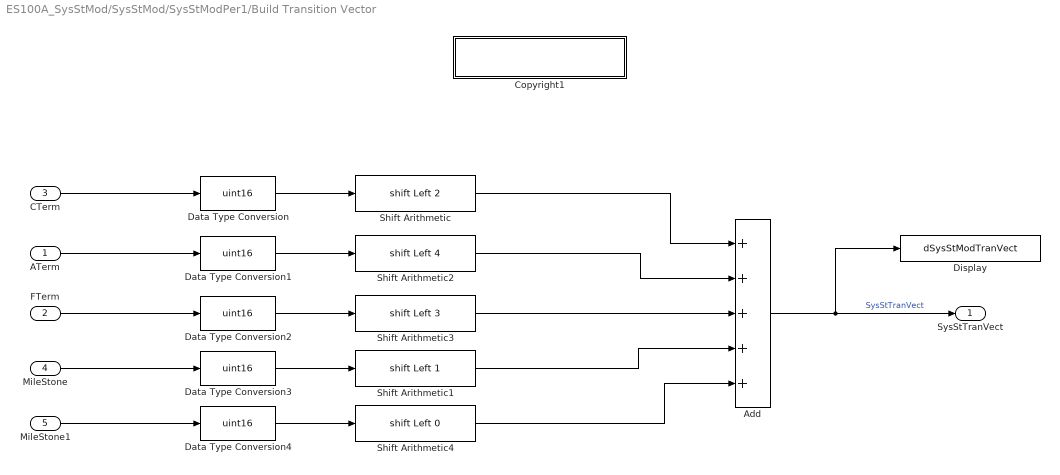
== system ES100A_SysStMod/SysStMod/SysStModPer1/Build Transition Vector ==
  ATerm : Inport
  FTerm : Inport  Port=2
  CTerm : Inport  Port=3
  MileStone : Inport  Port=4
  MileStone1 : Inport  Port=5
  Add : Sum  RequirementInfo={} %GIDa_03791183_2987_4e22_8003_9b45adce3860  Inputs=+++++
  Copyright1 : Subsystem  Description=|  mask(Copyright Information){none=on}
      | Copyright info block.                                               
      |                                                                     
      | Place copyright information at the top of every subsystem in design.
      mask prompts: none "No parameters"
      mask help: Place copyright information at the top of every subsystem in design.
      mask Display:
      | NxtrConf = 'Nexteer Confidential';
      | 
      | sys = bdroot; %handle for the current model ("system")
      | first = get_param(sys,'Created');
      | if(isempty(first))
      |     first = datestr(now,'yyyy');
      | else
      |     first = first(end-3:end);  %year is last four digits
      | end
      | 
      | last = get_param(sys,'LastModifiedDate');
      | if isempty(last)
      |     last = datestr(now,'yyyy');
      | else
      |     last = last(end-3:end);
      | end
      | 
      | if strcmp(first,last)
      |     fprintf('%s\nCopyright  %s Nexteer',NxtrConf,first);
      | else
      |     fprintf('%s\n%s%s-%s Nexteer',NxtrConf,char(169),first,last);
      | end
  Data Type Conversion{,1..4} (5 alike) : DataTypeConversion  OutDataTypeStr=uint16
  Display : DataStoreWrite  DataStoreName=dSysStModTranVect
  Shift Arithmetic : ArithShift  BitShiftNumber=2  BitShiftDirection=Left
  Shift Arithmetic1 : ArithShift  BitShiftNumber=1  BitShiftDirection=Left
  Shift Arithmetic2 : ArithShift  BitShiftNumber=4  BitShiftDirection=Left
  Shift Arithmetic3 : ArithShift  BitShiftNumber=3  BitShiftDirection=Left
  Shift Arithmetic4 : ArithShift  BitShiftDirection=Left
  SysStTranVect : Outport  RequirementInfo={'linktype_rmi_doors' '0000cf67 (/E-STEER Core/SubSystem Specifications/Electrical Actuator/Control Module/FDD Module Requirements/EA4/ES100A_SysStMod_1)' '#ES100A_53' 'true' 'REQ: ES100A_53' '' } %GIDa_13c09b51_3c72_4669_8720_9682c22482d8  InitialOutput=[8]
  wires:
  CTerm/1 -> Data Type Conversion/1
  Shift Arithmetic2/1 -> Add/2
  Shift Arithmetic3/1 -> Add/3
  Shift Arithmetic1/1 -> Add/4
  Shift Arithmetic/1 -> Add/1
  Add/1 -> SysStTranVect/1, Display/1  "SysStTranVect"
  Data Type Conversion/1 -> Shift Arithmetic/1
  Data Type Conversion1/1 -> Shift Arithmetic2/1
  Data Type Conversion2/1 -> Shift Arithmetic3/1
  Data Type Conversion3/1 -> Shift Arithmetic1/1
  ATerm/1 -> Data Type Conversion1/1
  FTerm/1 -> Data Type Conversion2/1
  MileStone/1 -> Data Type Conversion3/1
  MileStone1/1 -> Data Type Conversion4/1
  Data Type Conversion4/1 -> Shift Arithmetic4/1
  Shift Arithmetic4/1 -> Add/5

== system ES100A_SysStMod/SysStMod/SysStModPer1/Copyright1 ==

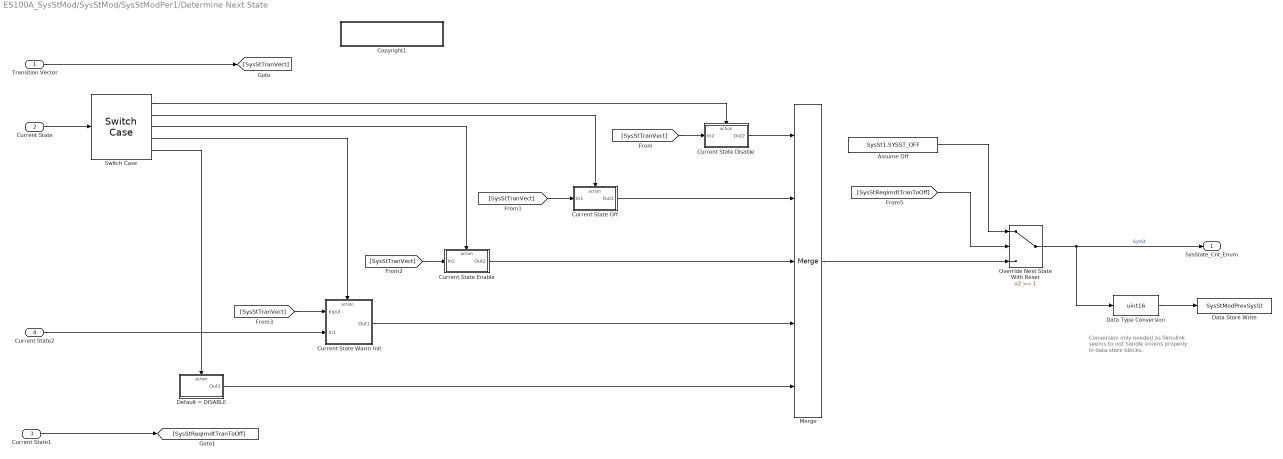
== system ES100A_SysStMod/SysStMod/SysStModPer1/Determine Next State ==
  note: Conversion only needed as Simulink
      | seems to not handle enums properly
      | in data store blocks.
  Transition Vector : Inport
  Current State : Inport  Port=2
  Current State1 : Inport  Port=3
  Current State2 : Inport  Port=4
  Assume Off : Constant  Value=SysSt1.SYSST_OFF
  Copyright1 : Subsystem  Description=|  mask(Copyright Information){none=on}
      | Copyright info block.                                               
      |                                                                     
      | Place copyright information at the top of every subsystem in design.
      mask prompts: none "No parameters"
      mask help: Place copyright information at the top of every subsystem in design.
      mask Display:
      | NxtrConf = 'Nexteer Confidential';
      | 
      | sys = bdroot; %handle for the current model ("system")
      | first = get_param(sys,'Created');
      | if(isempty(first))
      |     first = datestr(now,'yyyy');
      | else
      |     first = first(end-3:end);  %year is last four digits
      | end
      | 
      | last = get_param(sys,'LastModifiedDate');
      | if isempty(last)
      |     last = datestr(now,'yyyy');
      | else
      |     last = last(end-3:end);
      | end
      | 
      | if strcmp(first,last)
      |     fprintf('%s\nCopyright  %s Nexteer',NxtrConf,first);
      | else
      |     fprintf('%s\n%s%s-%s Nexteer',NxtrConf,char(169),first,last);
      | end
  Current State Disable : Subsystem  RequirementInfo={'linktype_rmi_doors' '0000cf67 (/E-STEER Core/SubSystem Specifications/Electrical Actuator/Control Module/FDD Module Requirements/EA4/ES100A_SysStMod_1)' '#ES100A_90' 'true' 'REQ: ES100A_90' '' ; 'linktype_rmi_doors' '0000cf67 (/E-STEER Core/SubSystem Specifications/Electrical Actuator/Control Module/FDD Module Requirements/EA4/ES100A_SysStMod_1)' '#ES100A_94' 'true' 'REQ: ES100A_94' '' } %GIDa_e1e50ad2_4789_4c4e_a4c7_002ffd1770da  TreatAsAtomicUnit=on
  Current State Enable : Subsystem  RequirementInfo={'linktype_rmi_doors' '0000cf67 (/E-STEER Core/SubSystem Specifications/Electrical Actuator/Control Module/FDD Module Requirements/EA4/ES100A_SysStMod_1)' '#ES100A_89' 'true' 'REQ: ES100A_89' '' } %GIDa_07685410_2e83_4a93_9d3f_b80ee72f3a0a  TreatAsAtomicUnit=on
  Current State Off : Subsystem  RequirementInfo={'linktype_rmi_doors' '0000cf67 (/E-STEER Core/SubSystem Specifications/Electrical Actuator/Control Module/FDD Module Requirements/EA4/ES100A_SysStMod_1)' '#ES100A_85' 'true' 'REQ: ES100A_85' '' } %GIDa_350cd354_659e_4f90_ac33_fd444e1467d6  TreatAsAtomicUnit=on
  Current State Warm Init : Subsystem  RequirementInfo={'linktype_rmi_doors' '0000cf67 (/E-STEER Core/SubSystem Specifications/Electrical Actuator/Control Module/FDD Module Requirements/EA4/ES100A_SysStMod_1)' '#ES100A_88' 'true' 'REQ: ES100A_88' '' ; 'linktype_rmi_doors' '0000cf67 (/E-STEER Core/SubSystem Specifications/Electrical Actuator/Control Module/FDD Module Requirements/EA4/ES100A_SysStMod_1)' '#ES100A_187' 'true' 'REQ: ES100A_187' '' ; 'linktype_rmi_doors' '0000cf67 (/E-STEER Core/SubSystem Specifications/Electrical Actuator/Control Module/FDD Module Requirements/EA4/ES100A_SysStMod_1)' '#ES100A_188' 'true' 'REQ: ES100A_188' '' } %GIDa_e2d8a05b_bdbd_4458_9f82_aa98d3940f68  TreatAsAtomicUnit=on
  Data Store Write : DataStoreWrite  DataStoreName=SysStModPrevSysSt
  Data Type Conversion : DataTypeConversion  OutDataTypeStr=uint16
  Default = DISABLE : Subsystem  RequirementInfo={'linktype_rmi_doors' '0000cf67 (/E-STEER Core/SubSystem Specifications/Electrical Actuator/Control Module/FDD Module Requirements/EA4/ES100A_SysStMod_1)' '#ES100A_99' 'true' 'REQ: ES100A_99' '' } %GIDa_105b2355_c427_4bb7_8494_107c3be44b57  TreatAsAtomicUnit=on
  Merge : Merge  Inputs=5
  Override Next State With Reset : Switch  RequirementInfo={'linktype_rmi_doors' '0000cf67 (/E-STEER Core/SubSystem Specifications/Electrical Actuator/Control Module/FDD Module Requirements/EA4/ES100A_SysStMod_1)' '#ES100A_91' 'true' 'REQ: ES100A_91' '' ; 'linktype_rmi_doors' '0000cf67 (/E-STEER Core/SubSystem Specifications/Electrical Actuator/Control Module/FDD Module Requirements/EA4/ES100A_SysStMod_1)' '#ES100A_92' 'true' 'REQ: ES100A_92' '' ; 'linktype_rmi_doors' '0000cf67 (/E-STEER Core/SubSystem Specifications/Electrical Actuator/Control Module/FDD Module Requirements/EA4/ES100A_SysStMod_1)' '#ES100A_93' 'true' 'REQ: ES100A_93' '' ; 'linktype_rmi_doors' '0000cf67 (/E-STEER Core/SubSystem Specifications/Electrical Actuator/Control Module/FDD Module Requirements/EA4/ES100A_SysStMod_1)' '#ES100A_96' 'true' 'REQ: ES100A_96' '' ; 'linktype_rmi_doors' '0000cf67 (/E-STEER Core/SubSystem Specifications/Electrical Actuator/Control Module/FDD Module Requirements/EA4/ES100A_SysStMod_1)' '#ES100A_97' 'true' 'REQ: ES100A_97' '' ; 'linktype_rmi_doors' '0000cf67 (/E-STEER Core/SubSystem Specifications/Electrical Actuator/Control Module/FDD Module Requirements/EA4/ES100A_SysStMod_1)' '#ES100A_98' 'true' 'REQ: ES100A_98' '' } %GIDa_d1dca712_56c2_4333_bc97_00cc09933cfa  Threshold=1  OutDataTypeStr=Enum: SysSt1
  Switch Case : SwitchCase  CaseConditions={SysSt1.SYSST_DI, SysSt1.SYSST_OFF, SysSt1.SYSST_ENA, SysSt1.SYSST_WRMININ}
  SysState_Cnt_Enum : Outport  InitialOutput=[3]
  wires:
  Current State/1 -> Switch Case/1
  Switch Case/1 -> Current State Disable/Action
  Transition Vector/1 -> [SysStTranVect]
  [SysStTranVect] -> Current State Disable/1(In2)
  [SysStTranVect] -> Current State Off/1(In1)
  [SysStTranVect] -> Current State Enable/1(In2)
  [SysStTranVect] -> Current State Warm Init/1(Input)
  Switch Case/5 -> Default = DISABLE/Action
  Current State Disable/1(Out2) -> Merge/1
  Current State Off/1(Out1) -> Merge/2
  Current State Enable/1(Out2) -> Merge/3
  Current State Warm Init/1(Out1) -> Merge/4
  Merge/1 -> Override Next State With Reset/3
  Assume Off/1 -> Override Next State With Reset/1
  [SysStReqImdtTranToOff] -> Override Next State With Reset/2
  Override Next State With Reset/1 -> Data Type Conversion/1, SysState_Cnt_Enum/1  "SysSt"
  Current State1/1 -> [SysStReqImdtTranToOff]
  Current State2/1 -> Current State Warm Init/2(In1)
  Default = DISABLE/1(Out1) -> Merge/5
  Switch Case/2 -> Current State Off/Action
  Switch Case/3 -> Current State Enable/Action
  Switch Case/4 -> Current State Warm Init/Action
  Data Type Conversion/1 -> Data Store Write/1

== system ES100A_SysStMod/SysStMod/SysStModPer1/Build Transition Vector/Copyright1 ==

== system ES100A_SysStMod/SysStMod/SysStModPer1/Determine Next State/Copyright1 ==

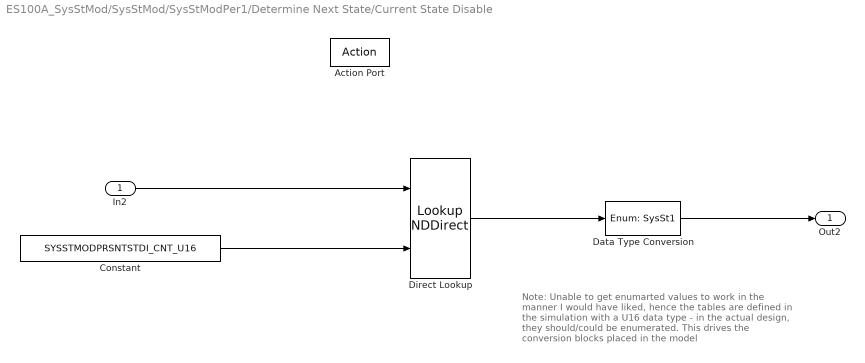
== system ES100A_SysStMod/SysStMod/SysStModPer1/Determine Next State/Current State Disable ==
  note: Note: Unable to get enumarted values to work in the
      | manner I would have liked, hence the tables are defined
      | in the simulation with a U16 data type - in the actual
      | design, they should/could be enumerated.  This drives
      |  the conversion blocks placed in the model
  In2 : Inport
  Action Port : ActionPort  ActionType=case
  Constant : Constant  Value=SYSSTMODPRSNTSTDI_CNT_U16
      settings: SamplingMode=Frame based
  Data Type Conversion : DataTypeConversion  OutDataTypeStr=Enum: SysSt1
  Direct Lookup : LookupNDDirect  NumberOfTableDimensions=1  TableIsInput=on
  Out2 : Outport
  wires:
  Direct Lookup/1 -> Data Type Conversion/1
  In2/1 -> Direct Lookup/1
  Constant/1 -> Direct Lookup/2
  Data Type Conversion/1 -> Out2/1

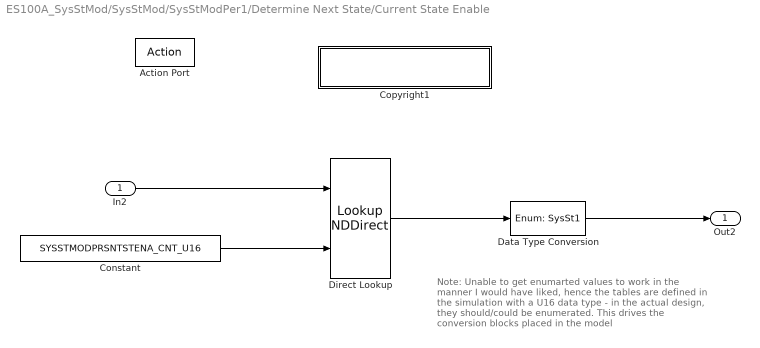
== system ES100A_SysStMod/SysStMod/SysStModPer1/Determine Next State/Current State Enable ==
  note: Note: Unable to get enumarted values to work in the
      | manner I would have liked, hence the tables are defined
      | in the simulation with a U16 data type - in the actual
      | design, they should/could be enumerated.  This drives
      |  the conversion blocks placed in the model
  In2 : Inport
  Action Port : ActionPort  ActionType=case
  Constant : Constant  Value=SYSSTMODPRSNTSTENA_CNT_U16
      settings: SamplingMode=Frame based
  Copyright1 : Subsystem  Description=|  mask(Copyright Information){none=on}
      | Copyright info block.                                               
      |                                                                     
      | Place copyright information at the top of every subsystem in design.
      mask prompts: none "No parameters"
      mask help: Place copyright information at the top of every subsystem in design.
      mask Display:
      | NxtrConf = 'Nexteer Confidential';
      | 
      | sys = bdroot; %handle for the current model ("system")
      | first = get_param(sys,'Created');
      | if(isempty(first))
      |     first = datestr(now,'yyyy');
      | else
      |     first = first(end-3:end);  %year is last four digits
      | end
      | 
      | last = get_param(sys,'LastModifiedDate');
      | if isempty(last)
      |     last = datestr(now,'yyyy');
      | else
      |     last = last(end-3:end);
      | end
      | 
      | if strcmp(first,last)
      |     fprintf('%s\nCopyright  %s Nexteer',NxtrConf,first);
      | else
      |     fprintf('%s\n%s%s-%s Nexteer',NxtrConf,char(169),first,last);
      | end
  Data Type Conversion : DataTypeConversion  OutDataTypeStr=Enum: SysSt1
  Direct Lookup : LookupNDDirect  NumberOfTableDimensions=1  TableIsInput=on
  Out2 : Outport
  wires:
  Direct Lookup/1 -> Data Type Conversion/1
  In2/1 -> Direct Lookup/1
  Constant/1 -> Direct Lookup/2
  Data Type Conversion/1 -> Out2/1

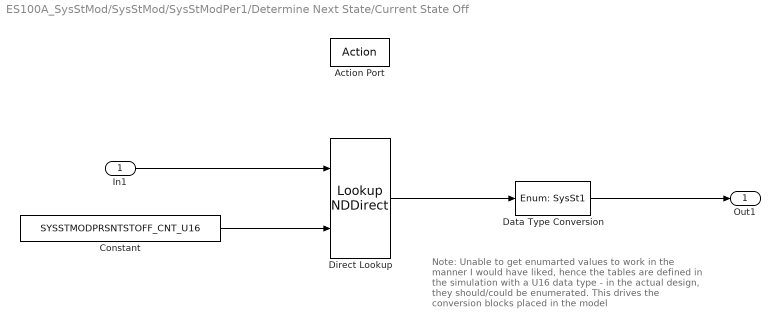
== system ES100A_SysStMod/SysStMod/SysStModPer1/Determine Next State/Current State Off ==
  note: Note: Unable to get enumarted values to work in the
      | manner I would have liked, hence the tables are defined
      | in the simulation with a U16 data type - in the actual
      | design, they should/could be enumerated.  This drives
      |  the conversion blocks placed in the model
  In1 : Inport
  Action Port : ActionPort  ActionType=case
  Constant : Constant  Value=SYSSTMODPRSNTSTOFF_CNT_U16
      settings: SamplingMode=Frame based
  Data Type Conversion : DataTypeConversion  OutDataTypeStr=Enum: SysSt1
  Direct Lookup : LookupNDDirect  NumberOfTableDimensions=1  TableIsInput=on
  Out1 : Outport
  wires:
  Direct Lookup/1 -> Data Type Conversion/1
  In1/1 -> Direct Lookup/1
  Constant/1 -> Direct Lookup/2
  Data Type Conversion/1 -> Out1/1

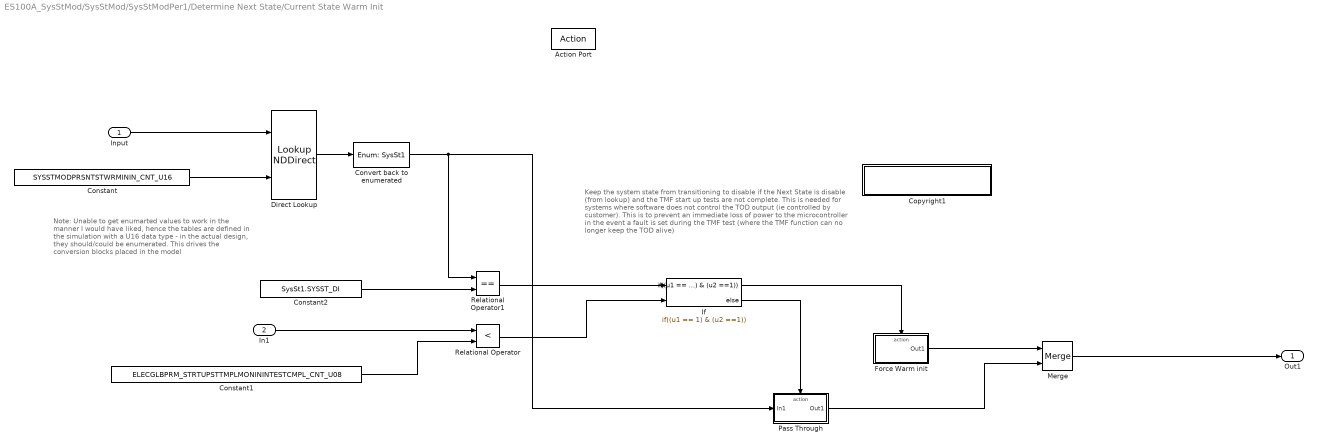
== system ES100A_SysStMod/SysStMod/SysStModPer1/Determine Next State/Current State Warm Init ==
  note: Note: Unable to get enumarted values to work in the
      | manner I would have liked, hence the tables are defined
      | in the simulation with a U16 data type - in the actual
      | design, they should/could be enumerated.  This drives
      |  the conversion blocks placed in the model
  note: Keep the system state from transitioning to disable if the
      | Next State is disable (from lookup) and the TMF start up tests
      | are not complete.
      | This is needed for systems where software does not control the TOD
      | output (ie controlled by customer).  This is to prevent an immediate loss
      | of power to the microcontroller in the event a fault is set during the TMF test
      | (where the TMF function can no longer keep the TOD alive)
  Input : Inport
  In1 : Inport  Port=2
  Action Port : ActionPort  ActionType=case
  Constant : Constant  Value=SYSSTMODPRSNTSTWRMININ_CNT_U16
      settings: SamplingMode=Frame based
  Constant1 : Constant  Value=ELECGLBPRM_STRTUPSTTMPLMONININTESTCMPL_CNT_U08
      settings: SamplingMode=Frame based
  Constant2 : Constant  Value=SysSt1.SYSST_DI
      settings: SamplingMode=Frame based
  Convert back to enumerated : DataTypeConversion  OutDataTypeStr=Enum: SysSt1
  Copyright1 : Subsystem  Description=|  mask(Copyright Information){none=on}
      | Copyright info block.                                               
      |                                                                     
      | Place copyright information at the top of every subsystem in design.
      mask prompts: none "No parameters"
      mask help: Place copyright information at the top of every subsystem in design.
      mask Display:
      | NxtrConf = 'Nexteer Confidential';
      | 
      | sys = bdroot; %handle for the current model ("system")
      | first = get_param(sys,'Created');
      | if(isempty(first))
      |     first = datestr(now,'yyyy');
      | else
      |     first = first(end-3:end);  %year is last four digits
      | end
      | 
      | last = get_param(sys,'LastModifiedDate');
      | if isempty(last)
      |     last = datestr(now,'yyyy');
      | else
      |     last = last(end-3:end);
      | end
      | 
      | if strcmp(first,last)
      |     fprintf('%s\nCopyright  %s Nexteer',NxtrConf,first);
      | else
      |     fprintf('%s\n%s%s-%s Nexteer',NxtrConf,char(169),first,last);
      | end
  Direct Lookup : LookupNDDirect  NumberOfTableDimensions=1  TableIsInput=on
  "Force Warm init " : Subsystem  TreatAsAtomicUnit=on
  If : If  RequirementInfo={'linktype_rmi_doors' '0000cf67 (/E-STEER Core/SubSystem Specifications/Electrical Actuator/Control Module/FDD Module Requirements/EA4/ES100A_SysStMod_1)' '#ES100A_95' 'true' 'REQ: ES100A_95' '' } %GIDa_abff26e5_d2fe_4d6b_8581_fd22b5a3a847  NumInputs=2  IfExpression=(u1 == 1) & (u2 ==1)
  Merge : Merge
  Pass Through : Subsystem  TreatAsAtomicUnit=on
  Relational Operator : RelationalOperator  Operator=<  OutDataTypeStr=boolean
  Relational Operator1 : RelationalOperator  Operator===  OutDataTypeStr=boolean
  Out1 : Outport
  wires:
  Direct Lookup/1 -> Convert back to enumerated/1
  If/1 -> "Force Warm init "/Action
  "Force Warm init "/1(Out1) -> Merge/1
  Merge/1 -> Out1/1
  If/2 -> Pass Through/Action
  Input/1 -> Direct Lookup/1
  In1/1 -> Relational Operator/1
  Constant/1 -> Direct Lookup/2
  Constant1/1 -> Relational Operator/2
  Relational Operator/1 -> If/2
  Pass Through/1(Out1) -> Merge/2
  Convert back to enumerated/1 -> Pass Through/1(In1), Relational Operator1/1
  Constant2/1 -> Relational Operator1/2
  Relational Operator1/1 -> If/1

== system ES100A_SysStMod/SysStMod/SysStModPer1/Determine Next State/Default = DISABLE ==
  Action Port : ActionPort  ActionType=default
  Constant : Constant  Value=SysSt1.SYSST_DI
  Out1 : Outport
  wires:
  Constant/1 -> Out1/1

== system ES100A_SysStMod/SysStMod/SysStModPer1/Determine Next State/Current State Enable/Copyright1 ==

== system ES100A_SysStMod/SysStMod/SysStModPer1/Determine Next State/Current State Warm Init/Copyright1 ==

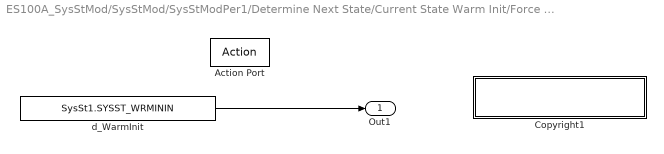
== system ES100A_SysStMod/SysStMod/SysStModPer1/Determine Next State/Current State Warm Init/Force Warm init  ==
  Action Port : ActionPort  ActionType=then
  Copyright1 : Subsystem  Description=|  mask(Copyright Information){none=on}
      | Copyright info block.                                               
      |                                                                     
      | Place copyright information at the top of every subsystem in design.
      mask prompts: none "No parameters"
      mask help: Place copyright information at the top of every subsystem in design.
      mask Display:
      | NxtrConf = 'Nexteer Confidential';
      | 
      | sys = bdroot; %handle for the current model ("system")
      | first = get_param(sys,'Created');
      | if(isempty(first))
      |     first = datestr(now,'yyyy');
      | else
      |     first = first(end-3:end);  %year is last four digits
      | end
      | 
      | last = get_param(sys,'LastModifiedDate');
      | if isempty(last)
      |     last = datestr(now,'yyyy');
      | else
      |     last = last(end-3:end);
      | end
      | 
      | if strcmp(first,last)
      |     fprintf('%s\nCopyright  %s Nexteer',NxtrConf,first);
      | else
      |     fprintf('%s\n%s%s-%s Nexteer',NxtrConf,char(169),first,last);
      | end
  d_WarmInit : Constant  Value=SysSt1.SYSST_WRMININ
  Out1 : Outport  OutDataTypeStr=Enum: SysSt1  InitialOutput=[SysSt1.SYSST_WRMININ]
  wires:
  d_WarmInit/1 -> Out1/1

== system ES100A_SysStMod/SysStMod/SysStModPer1/Determine Next State/Current State Warm Init/Pass Through ==
  In1 : Inport
  Action Port : ActionPort  ActionType=else
  Copyright1 : Subsystem  Description=|  mask(Copyright Information){none=on}
      | Copyright info block.                                               
      |                                                                     
      | Place copyright information at the top of every subsystem in design.
      mask prompts: none "No parameters"
      mask help: Place copyright information at the top of every subsystem in design.
      mask Display:
      | NxtrConf = 'Nexteer Confidential';
      | 
      | sys = bdroot; %handle for the current model ("system")
      | first = get_param(sys,'Created');
      | if(isempty(first))
      |     first = datestr(now,'yyyy');
      | else
      |     first = first(end-3:end);  %year is last four digits
      | end
      | 
      | last = get_param(sys,'LastModifiedDate');
      | if isempty(last)
      |     last = datestr(now,'yyyy');
      | else
      |     last = last(end-3:end);
      | end
      | 
      | if strcmp(first,last)
      |     fprintf('%s\nCopyright  %s Nexteer',NxtrConf,first);
      | else
      |     fprintf('%s\n%s%s-%s Nexteer',NxtrConf,char(169),first,last);
      | end
  Out1 : Outport
  wires:
  In1/1 -> Out1/1

== system ES100A_SysStMod/SysStMod/SysStModPer1/Determine Next State/Current State Warm Init/Force Warm init /Copyright1 ==

== system ES100A_SysStMod/SysStMod/SysStModPer1/Determine Next State/Current State Warm Init/Pass Through/Copyright1 ==
